simulink model "ARM_2DOF_Step_Response"  (R2021a)
settings: Solver=VariableStepAuto  StartTime=0.0  StopTime=20  RelTol=1e-5
settings Model: SimulationMode=accelerator  Creator=Zicx  LastModifiedBy=Zicx
settings SolverCC: MaxConsecutiveZCs=1500  ZeroCrossAlgorithm=Adaptive

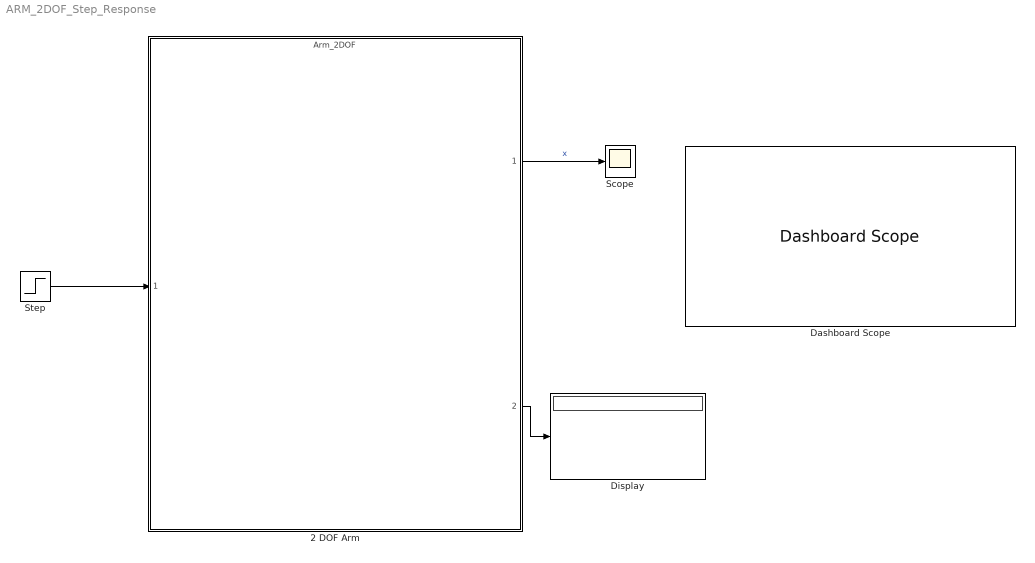
== system ARM_2DOF_Step_Response ==
  2 DOF Arm : ModelReference  ModelNameDialog=Arm_2DOF  SimulationMode=Normal  ModelReferenceVersion=1.48
  Dashboard Scope : DashboardScope
  Display : Display
  Scope : Scope
  Step : Step  After=[1;1]  SampleTime=0
  wires:
  Step/1 -> 2 DOF Arm/1
  2 DOF Arm/1 -> Scope/1  "x"
  2 DOF Arm/2 -> Display/1
